simulink model "rtwdemo_abstime"  (Simulink 6.0)
settings: Solver=FixedStepDiscrete  StartTime=0.0  StopTime=10.0  RelTol=1e-3
undefined symbols (not defined in the file or in its folder): DiscIntNeverNeededParam
libraries: rtwdemowidgets x2, simulink x1
settings Model: Creator=The MathWorks Inc.  LastModifiedBy=batserve  ExtModeAutoUpdateStatusClock=off
settings DataIOCC: SaveOutput=off  SaveTime=off  SignalLoggingName=logsOut
settings OptimizationCC: InlineParams=on  EnforceIntegerDowncast=off  StateBitsets=on  DataBitsets=on  UseTempVars=on
settings DebuggingCC: CheckExecutionContextPreStartOutputMsg=on  CheckExecutionContextRuntimeOutputMsg=on
settings RTWCC: TLCOptions=-p0 -aWarnNonSaturatedBlocks=0  Description=RTW Embedded Coder (no auto configuration)  GenerateReport=on  RTWVerbose=off  ProcessScript=grt_make_rtw_hook  LaunchReport=on
settings CodeAppCC: ForceParamTrailComments=on
settings GRTTargetCC: MatFileLogging=off

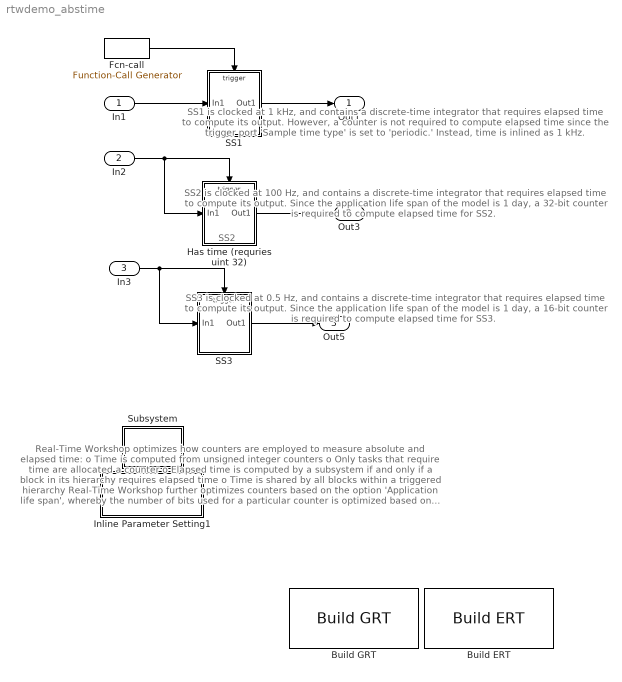
== system rtwdemo_abstime ==
  note: Real-Time Workshop optimizes how counters are employed to measure absolute and elapsed time:
      |
      | o Time is computed from unsigned integer counters
      | o Only tasks that require time are allocated a counter
      | o Elapsed time is computed by a subsystem if and only if a block in its hierarchy requires elapsed time
      | o Time is shared by all blocks within a triggered hierarchy
      |
      | Real-Time Workshop further optimizes counters based on the option 'Application life span', whereby
      | the number of bits used for a particular counter is optimized based on how long the application
      | will run.
  note: SS1 is clocked at 1 kHz, and contains a discrete-time integrator that requires
      | elapsed time to compute its output.  However, a counter is not required to
      | compute elapsed time since the trigger port 'Sample time type' is set to
      | 'periodic.'  Instead, time is inlined as 1 kHz.
  note: SS2 is clocked at 100 Hz, and contains a discrete-time integrator that requires
      | elapsed time to compute its output.  Since the application life span of the model
      | is 1 day, a 32-bit counter is required to compute elapsed time for SS2.
  note: SS3 is clocked at 0.5 Hz, and contains a discrete-time integrator that requires
      | elapsed time to compute its output.  Since the application life span of the model
      | is 1 day, a 16-bit counter is required to compute elapsed time for SS3.
  note: SS2
  In1 : Inport  Port=1  LatchInput=off
  In2 : Inport  Port=2  SampleTime=.01  LatchInput=off
  In3 : Inport  Port=3  SampleTime=2  LatchInput=off
  Build ERT : rtwdemowidgets/Build ERT  attrib_overrides={}
  Build GRT : rtwdemowidgets/Build GRT  attrib_overrides={}
  Fcn-call : simulink/Ports & Subsystems/Function-Call Generator  sample_time=0.001  numberOfIterations=1
  Has time (requries uint 32) : Subsystem  PropExecContextAcrossSSBoundary=on
  Inline Parameter Setting1 : Subsystem  Orientation=up  PropExecContextAcrossSSBoundary=on
      settings: OpenFcn=m=get_param(bdroot,'name'); eval([m,'([],[],[],''compile'');']); eval([m,'([],[],[],''term'');']);
      mask Display: disp(sprintf('Display Sample\nTime Colors\n(double-click)'))
  SS1 : Subsystem  PropExecContextAcrossSSBoundary=on
  SS3 : Subsystem  PropExecContextAcrossSSBoundary=on
  Subsystem : Subsystem  PropExecContextAcrossSSBoundary=on
      mask Display: disp(['Did you\nknow ..','.'])
  Out1 : Outport
  Out3 : Outport  Port=2
  Out5 : Outport  Port=3
  wires:
  In1/1 -> SS1/1(In1)
  SS1/1(Out1) -> Out1/1
  Fcn-call/1 -> SS1/Trigger
  Has time (requries uint 32)/1(Out1) -> Out3/1
  In2/1 -> Has time (requries uint 32)/Trigger, Has time (requries uint 32)/1(In1)
  SS3/1(Out1) -> Out5/1
  In3/1 -> SS3/Trigger, SS3/1(In1)

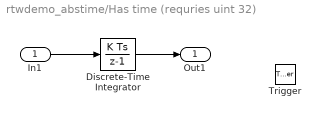
== system rtwdemo_abstime/Has time (requries uint 32) ==
  In1 : Inport  Port=1  LatchInput=off
  Trigger : TriggerPort  TriggerType=either  SampleTime=-1
  Discrete-Time Integrator : DiscreteIntegrator  SampleTime=-1  ICPrevOutput=DiscIntNeverNeededParam  ICPrevScaledInput=DiscIntNeverNeededParam
  Out1 : Outport  InitialOutput=0
  wires:
  Discrete-Time Integrator/1 -> Out1/1
  In1/1 -> Discrete-Time Integrator/1

== system rtwdemo_abstime/Inline Parameter Setting1 ==

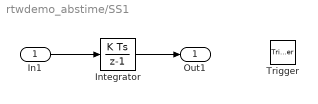
== system rtwdemo_abstime/SS1 ==
  In1 : Inport  Port=1  LatchInput=off
  Trigger : TriggerPort  TriggerType=function-call  SampleTimeType=periodic  SampleTime=0.001
  Integrator : DiscreteIntegrator  SampleTime=-1  ICPrevOutput=DiscIntNeverNeededParam  ICPrevScaledInput=DiscIntNeverNeededParam
  Out1 : Outport  InitialOutput=0
  wires:
  In1/1 -> Integrator/1
  Integrator/1 -> Out1/1

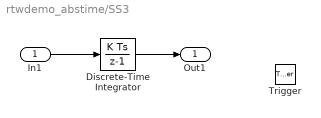
== system rtwdemo_abstime/SS3 ==
  In1 : Inport  Port=1  LatchInput=off
  Trigger : TriggerPort  TriggerType=either
  Discrete-Time Integrator : DiscreteIntegrator  SampleTime=-1  ICPrevOutput=DiscIntNeverNeededParam  ICPrevScaledInput=DiscIntNeverNeededParam
  Out1 : Outport  InitialOutput=0
  wires:
  In1/1 -> Discrete-Time Integrator/1
  Discrete-Time Integrator/1 -> Out1/1

== system rtwdemo_abstime/Subsystem ==
  note: Assume an unsigned integer counter is incrementing at 1 kHz.  The number
      | of bits required to avoid an integer overflow is as follows:
      |
      | Time span < 0.25 sec :  8-bits
      | Time span < 1 min:       16-bits
      | Time span < 49 days:    32-bits
      | Time span > 50 days:    64-bits
      |
      | And, the 64-bit timer will not overflow for 590 million years!
      |
      | Leveraging the 'Application life span' option provided by Simulink allows you to
      | avoid timer overflows efficiently without wasting memory.
